simulink model "simulate_battery_wo_cap"  (R2021a)
settings: Solver=VariableStepAuto  StartTime=0.0  StopTime=time_val  RelTol=1e-3
settings Model: Creator=saleh  LastModifiedBy=saleh

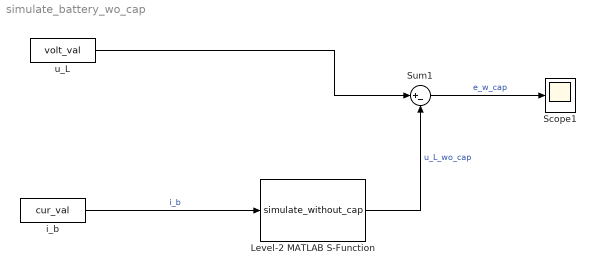
== system simulate_battery_wo_cap ==
  Level-2 MATLAB S-Function : M-S-Function  FunctionName=simulate_without_cap  Parameters=x_conv, a, Qe
  Scope1 : Scope
  Sum1 : Sum  Inputs=|+-
  i_b : FromWorkspace  VariableName=cur_val
  u_L : FromWorkspace  VariableName=volt_val
  wires:
  i_b/1 -> Level-2 MATLAB S-Function/1  "i_b"
  u_L/1 -> Sum1/1
  Level-2 MATLAB S-Function/1 -> Sum1/2  "u_L_wo_cap"
  Sum1/1 -> Scope1/1  "e_w_cap"
